simulink model "calcul_phi_vy_vx"  (R2024b)
settings: Solver=FixedStepAuto  StartTime=0.0  StopTime=10.0  FixedStep=Ts  RelTol=1e-3
values from neighbouring files (symbols this model uses):
  v0 = 10    [getItRunning.m]
undefined symbols (not defined in the file or in its folder): gyro, Izz, m, Ts
settings Model: Creator=marti  LastModifiedBy=marti

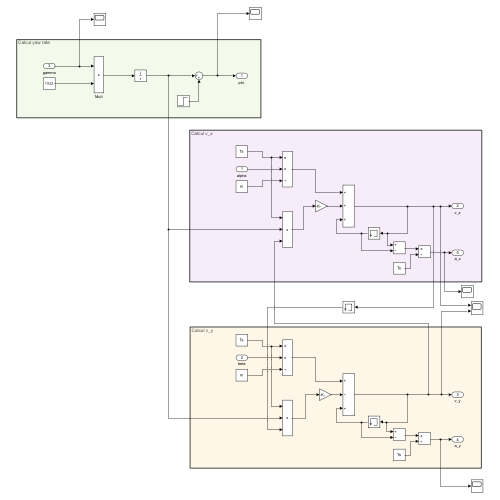
[thumbnail: Simulink's stored preview of the top-level diagram]
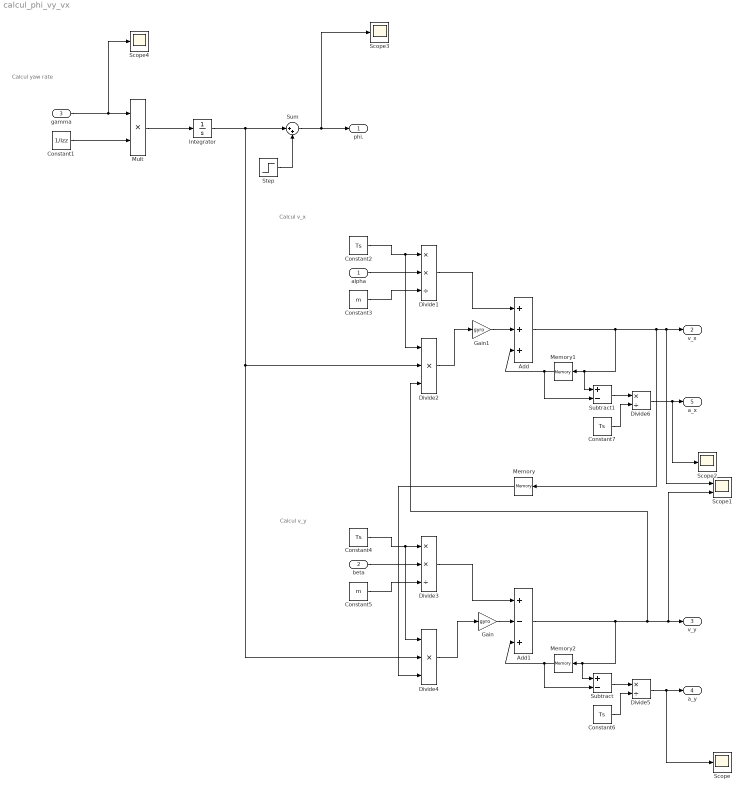
== system calcul_phi_vy_vx ==
  note: Calcul v_y
  note: Calcul v_x
  note: Calcul yaw rate
  alpha : Inport
  beta : Inport  Port=2
  gamma : Inport  Port=3
  Add : Sum  Inputs=+++
  Add1 : Sum  Inputs=+-+
  Constant1 : Constant  Value=1/Izz
  Constant{2,4,6..7} (4 alike) : Constant  Value=Ts
  Constant3 : Constant  Value=m
  Constant5 : Constant  Value=m
  Divide1 : Product  Inputs=**/
  Divide2 : Product  Inputs=***
  Divide3 : Product  Inputs=**/
  Divide4 : Product  Inputs=***
  Divide5 : Product  Inputs=*/
  Divide6 : Product  Inputs=*/
  Gain : Gain  Gain=gyro
  Gain1 : Gain  Gain=gyro
  Integrator : Integrator
  Memory : Memory  InitialCondition=v0
  Memory1 : Memory  InitialCondition=v0
  Memory2 : Memory
  Mult : Product  Inputs=**
  Scope{,2..4} (4 alike) : Scope
  Scope1 : Scope  NumInputPorts=2
  Step : Step  Time=3  After=0  SampleTime=0
  Subtract : Sum  Inputs=+-
  Subtract1 : Sum  Inputs=+-
  Sum : Sum  Inputs=|++
  phi. : Outport
  v_x : Outport  Port=2
  v_y : Outport  Port=3
  a_y : Outport  Port=4
  a_x : Outport  Port=5
  wires:
  gamma/1 -> Scope4/1, Mult/1
  Constant1/1 -> Mult/2
  Mult/1 -> Integrator/1
  alpha/1 -> Divide1/2
  Constant2/1 -> Divide2/1, Divide1/1
  Constant3/1 -> Divide1/3
  Divide1/1 -> Add/1
  Memory2/1 -> Subtract/2, Add1/3
  Divide3/1 -> Add1/1
  Constant5/1 -> Divide3/3
  Constant4/1 -> Divide4/1, Divide3/1
  Add1/1 -> Divide2/3, Scope1/2, v_y/1, Subtract/1, Memory2/1
  beta/1 -> Divide3/2
  Subtract/1 -> Divide5/1
  Constant6/1 -> Divide5/2
  Divide5/1 -> Scope/1, a_y/1
  Divide6/1 -> Scope2/1, a_x/1
  Subtract1/1 -> Divide6/1
  Memory1/1 -> Subtract1/2, Add/3
  Constant7/1 -> Divide6/2
  Gain/1 -> Add1/2
  Divide4/1 -> Gain/1
  Gain1/1 -> Add/2
  Divide2/1 -> Gain1/1
  Integrator/1 -> Sum/1, Divide2/2, Divide4/2
  Add/1 -> Subtract1/1, Memory1/1, Memory/1, Scope1/1, v_x/1
  Memory/1 -> Divide4/3
  Step/1 -> Sum/2
  Sum/1 -> Scope3/1, phi./1
